simulink model "simulacao"  (Simulink 6.0)
settings: Solver=ode45  StartTime=0.0  StopTime=10.0  RelTol=1e-3
settings Model: LastModifiedBy=aluno

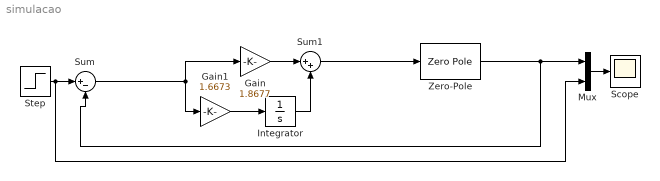
== system simulacao ==
  Gain : Gain  Gain=1.8677
  Gain1 : Gain  Gain=1.6673
  Integrator : Integrator
  Mux : Mux  Inputs=2
  Scope : Scope
  Step : Step  SampleTime=0
  Sum : Sum  Inputs=|+-
  Sum1 : Sum  Inputs=|++
  Zero-Pole : ZeroPole  Zeros=[-10]  Poles=[-8 -8 0.5]  Gain=10
  wires:
  Zero-Pole/1 -> Sum/2, Mux/1
  Step/1 -> Sum/1, Mux/2
  Gain/1 -> Sum1/1
  Integrator/1 -> Sum1/2
  Gain1/1 -> Integrator/1
  Sum1/1 -> Zero-Pole/1
  Sum/1 -> Gain/1, Gain1/1
  Mux/1 -> Scope/1
